simulink model "Dec_10_updated_33_bus_system_2MW_DG"  (R2023a)
settings: Solver=FixedStepAuto  StartTime=0.0  StopTime=0.3  RelTol=1e-3  EnableMultiTasking=on
undefined symbols (not defined in the file or in its folder): D1, Delta, DiscIntNeverNeededParam, Ts, Ts_Power
libraries: spsSeriesRLCBranchLib x42, spsThreePhaseVIMeasurementLib x35, spsThreePhaseSeriesRLCBranchLib x33, spsLoadFlowBusLib x33, spsThreePhaseParallelRLCLoadLib x31, simulink x8, spsMeanLib x5, spsFirstOrderFilterLib x4, spsStairGeneratorLib x3, spsBoostConverterLib x2, spsPowerPositiveSequenceLib x2, spsabctodq0Lib x2
(part 2 of 3)

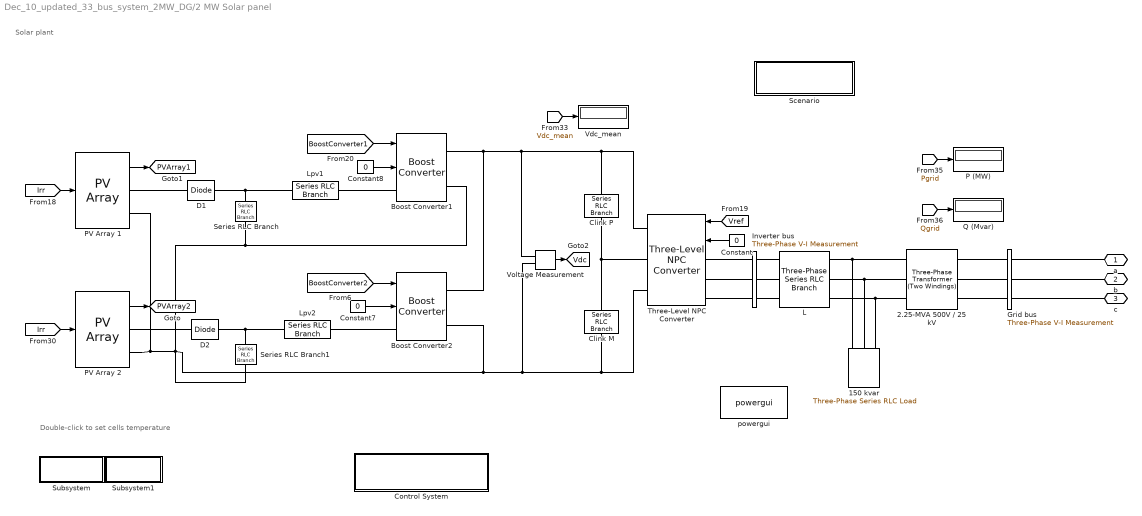
== system Dec_10_updated_33_bus_system_2MW_DG/2 MW Solar panel ==
  note: Solar plant
  note: Double-click to set cells temperature
  150 kvar : spsThreePhaseSeriesRLCLoadLib/Three-Phase Series RLC Load  LConnTagsString=A|B|C  Configuration=Y (grounded)  NominalVoltage=500  Vabc=[1e3 1e3 1e3]  Vabcp=[1e3 1e3 1e3]  NominalFrequency=50  UnbalancedPower=off  ActivePower=3000  InductivePower=0  CapacitivePower=150000  Pabc=[10e3 9e3 11e3]  QLabc=[100 90 110]  QCabc=[100 90 110]  Pabcp=[10e3 9e3 11e3]  QLabcp=[100 90 110]  QCabcp=[100 90 110]  Measurements=None  LoadType=constant Z
  2.25-MVA 500V / 25 kV : spsThreePhaseTransformerTwoWindingsLib/Three-Phase Transformer (Two Windings)  Winding1Connection=Yg  Winding2Connection=Delta (D1)  CoreType=Three single-phase transformers  SetSaturation=off  Hysteresis=off  DataFile='hysteresis'  SetInitialFlux=off  Measurements=None  UNITS=pu  NominalPower=[2.25e6 , 50 ]  Winding1=[ 33e3 , 0.001 , 0.03 ]  Winding2=[500 , 0.001 , 0.03 ]  Rm=200  Lm=200  L0=0.5  Saturation=[ 0,0 ; 0.0024,1.2 ; 1.0,1.52 ]  InitialFluxes=[ 0.8 , -0.8 , 0.7 ]  BreakLoop=off  DiscreteSolver=Trapezoidal iterative  DataType=off  TransfoNumber=0
  Boost Converter1 : spsBoostConverterLib/Boost Converter  ModelType=Switching devices  Ron=1e-4  Rs=1e6  Cs=inf  Vforward=[0,0]  Ron_Diode=1e-4  Rs_Diode=1e6  Cs_Diode=inf  Vf_Diode=0  Rs_CurrentSource=inf  Ron_ACsource=1e-3
      settings: LibrarySourceBlock=sps_lib/Power Electronics/Boost Converter
  Boost Converter2 : spsBoostConverterLib/Boost Converter  ModelType=Switching devices  Ron=1e-4  Rs=1e6  Cs=inf  Vforward=[0,0]  Ron_Diode=1e-4  Rs_Diode=1e6  Cs_Diode=inf  Vf_Diode=0  Rs_CurrentSource=inf  Ron_ACsource=1e-3
      settings: LibrarySourceBlock=sps_lib/Power Electronics/Boost Converter
  Clink M : spsSeriesRLCBranchLib/Series RLC Branch  LConnTagsString=__new0  RConnTagsString=__new0  BranchType=C  Resistance=1e-6  Inductance=1e-3  SetiL0=off  InitialCurrent=0  Capacitance=150e-3  Setx0=on  InitialVoltage=500  Measurements=None
  Clink P : spsSeriesRLCBranchLib/Series RLC Branch  LConnTagsString=__new0  RConnTagsString=__new0  BranchType=C  Resistance=1e-6  Inductance=1e-3  SetiL0=off  InitialCurrent=0  Capacitance=150e-3  Setx0=on  InitialVoltage=500  Measurements=None
  Constant : Constant  Value=0  SampleTime=Ts
  Constant7 : Constant  Value=0  SampleTime=Ts
  Constant8 : Constant  Value=0  SampleTime=Ts
  Control System : Subsystem
      mask Display: disp('CONTROL SYSTEM')
  D1 : spsDiodeLib/Diode  Ron=1e-4  Lon=0  Vf=0  IC=0  UseSnubber=0  Rs=1e6  Cs=inf  Measurements=off
  D2 : spsDiodeLib/Diode  Ron=1e-4  Lon=0  Vf=0  IC=0  UseSnubber=0  Rs=1e6  Cs=inf  Measurements=off
  Grid bus : spsThreePhaseVIMeasurementLib/Three-Phase V-I Measurement  VoltageMeasurement=phase-to-ground  SetLabelV=on  LabelV=Vgrid  Vpu=off  VpuLL=off  CurrentMeasurement=yes  SetLabelI=on  LabelI=Igrid  Ipu=off  Pbase=100e6  Vbase=500e3  OutputType=Magnitude  PhasorSimulation=off  PSBequivalent=0
  Inverter bus : spsThreePhaseVIMeasurementLib/Three-Phase V-I Measurement  VoltageMeasurement=phase-to-phase  SetLabelV=on  LabelV=Vinv  Vpu=off  VpuLL=off  CurrentMeasurement=no  SetLabelI=off  LabelI=Iabc_B1  Ipu=off  Pbase=100e6  Vbase=500e3  OutputType=Magnitude  PhasorSimulation=off  PSBequivalent=0
  L : spsThreePhaseSeriesRLCBranchLib/Three-Phase Series RLC Branch  LConnTagsString=A|B|C  RConnTagsString=A|B|C  BranchType=RL  Resistance=1e-3  Inductance=44.2e-6  Capacitance=inf  Measurements=None
  Lpv1 : spsSeriesRLCBranchLib/Series RLC Branch  LConnTagsString=__new0  RConnTagsString=__new0  BranchType=RL  Resistance=1e-3  Inductance=1e-3  SetiL0=off  InitialCurrent=0  Capacitance=120e-3  Setx0=off  InitialVoltage=0  Measurements=None
  Lpv2 : spsSeriesRLCBranchLib/Series RLC Branch  LConnTagsString=__new0  RConnTagsString=__new0  BranchType=RL  Resistance=1e-3  Inductance=1e-3  SetiL0=off  InitialCurrent=0  Capacitance=120e-3  Setx0=off  InitialVoltage=0  Measurements=None
  P (MW) : Display
      settings: Format=bank  Decimation=200
  PV Array 1 : spsPVArrayLib/PV Array  Npar=282  Nser=15  PlotType=array @ 1000 W/m2 & specified temperatures  S_vec=[ 1000 250]  Temp_C_vec="[ 45 25  ]"  ModuleName=User-defined  PlotWhenSelected=off  Pm=355.012  Ncell=83  Voc=51.9  Isc=8.68  Vm=43.4  Im=8.18  beta_Voc_pc=-0.304  alpha_Isc_pc=0.017  beta_Voc=-0.15778  alpha_Isc=0.0014756  IL=8.6865  I0=3.3093e-11  nI=0.92618  Rsh=389.4331  Rs=0.29289  RobustModel=on  RobustCellTemperature=25  BAL=on  Tc=1e-6  Tfilter=5e-5
      settings: AttributesFormatString=(%<RobustCellTemperature> deg. C)
  PV Array 2 : spsPVArrayLib/PV Array  Npar=122  Nser=14  PlotType=array @ 1000 W/m2 & specified temperatures  S_vec=[ 1000 250]  Temp_C_vec="[ 45 25  ]"  ModuleName=User-defined  PlotWhenSelected=off  Pm=293.664  Ncell=60  Voc=39.5  Isc=9.60  Vm=32.2  Im=9.12  beta_Voc_pc=-0.300  alpha_Isc_pc=0.03  beta_Voc=-0.1185  alpha_Isc=0.00288  IL=9.6627  I0=3.1923e-11  nI=0.96973  Rsh=336.4947  Rs=0.3029  RobustModel=on  RobustCellTemperature=25  BAL=on  Tc=1e-6  Tfilter=5e-5
      settings: AttributesFormatString=(%<RobustCellTemperature> deg. C)
  Q (Mvar) : Display
      settings: Format=bank  Decimation=200
  Scenario : Subsystem
      mask Display: disp('Scenario & Scopes')
  Series RLC Branch : spsSeriesRLCBranchLib/Series RLC Branch  LConnTagsString=__new0  RConnTagsString=__new0  BranchType=C  Resistance=1  Inductance=1e-3  SetiL0=off  InitialCurrent=0  Capacitance=200e-6  Setx0=on  InitialVoltage=650  Measurements=None
  Series RLC Branch1 : spsSeriesRLCBranchLib/Series RLC Branch  LConnTagsString=__new0  RConnTagsString=__new0  BranchType=C  Resistance=1  Inductance=1e-3  SetiL0=off  InitialCurrent=0  Capacitance=200e-6  Setx0=on  InitialVoltage=450  Measurements=None
  Subsystem : Subsystem
      settings: OpenFcn=|
      | SystemName1=gcs;
      | BlockName1=[SystemName1, '/', 'PV Array 1'];
      | set_param(BlockName1,'RobustCellTemperature','25');
      | set_param(BlockName1,'ForegroundColor','black');
      | BlockName2=[SystemName1, '/', 'PV Array 2'];
      | set_param(BlockName2,'RobustCellTemperature','25');
      | set_param(BlockName2,'ForegroundColor','black');
      mask Display: disp('25 deg. C')
  Subsystem1 : Subsystem
      settings: OpenFcn=|
      | SystemName1=gcs;
      | BlockName1=[SystemName1, '/', 'PV Array 1'];
      | set_param(BlockName1,'RobustCellTemperature','45');
      | set_param(BlockName1,'ForegroundColor','red');
      | BlockName2=[SystemName1, '/', 'PV Array 2'];
      | set_param(BlockName2,'RobustCellTemperature','45');
      | set_param(BlockName2,'ForegroundColor','red');
      mask Display: disp('45 deg. C')
  Three-Level NPC Converter : spsThreeLevelNPCConverterLib/Three-Level NPC Converter  ModelType=Switching devices  Ron=1e-4/2  Rs=1e6  Cs=inf  Vforward=[0,0]  Ron_Diode=1e-4  Rs_Diode=1e6  Cs_Diode=inf  Vf_Diode=0  Rs_CurrentSource=inf  Ron_ACsource=1e-3
      settings: LibrarySourceBlock=|
      | sps_lib/Power Electronics/Three-Level
      | NPC Converter
  Vdc_mean : Display
      settings: Decimation=200
  Voltage Measurement : spsVoltageMeasurementLib/Voltage Measurement  PhasorSimulation=off  OutputType=Complex  PSBequivalent=0
  powergui : spspowerguiLib/powergui  Priority=2  SimulationMode=Discrete  SampleTime=Ts_Power  frequency=60  Iterations=50  frequencyindice=0  Pbase=100e6  ErrMax=1e-4  UnitsV=kV  UnitsW=MW  buscounter=0  FunctionMessages=off  echomessages=off  EnableUseOfTLC=off  CurrentSourceSwitches=off  DisableSnubberDevices=off  DisableRonSwitches=off  DisableVfSwitches=off  DisplayEquations=off  AutomaticDiscreteSolvers=off  SolverType=Tustin/Backward Euler (TBE)  Interpol=off  ExternalGateDelay=off  methode=off  Ts=0  x0status=blocks  SPID=off  SwTol=0  HookPort=off  NonlinearTolerance=1e-4  nMaxIteration=100  ContinueOnMaxIteration=on  RestoreLinks=warning  ResistiveCurrentMeasurement=off  Frange=[0:2:500]  Ylog=off  Xlog=off  ShowGrid=off  save=off  variable=ZData  structure=Scope_VIgrid  ZoomFFT=off  StartTime=0.18  cycles=1  DisplayStyle=1  fundamental=60  FreqAxis=on  MaxFrequency=3500  frequencyindicesteady=1  RmsSteady=1  display=off
  a : PMIOPort  Side=Right
  b : PMIOPort  Port=2  Side=Right
  c : PMIOPort  Port=3  Side=Right
  tag scope: PVArray1=global, PVArray2=global, Vdc=global
  wires:
  [Pgrid] -> P (MW)/1
  Constant7/1 -> Boost Converter2/2
  Constant8/1 -> Boost Converter1/2
  PV Array 2/1 -> [PVArray2]
  PV Array 1/1 -> [PVArray1]
  [Irr] -> PV Array 2/1
  [BoostConverter1] -> Boost Converter1/1
  Constant/1 -> Three-Level NPC Converter/2
  [Vdc_mean] -> Vdc_mean/1
  [Vref] -> Three-Level NPC Converter/1
  [BoostConverter2] -> Boost Converter2/1
  Voltage Measurement/1 -> [Vdc]
  [Qgrid] -> Q (Mvar)/1
  [Irr] -> PV Array 1/1
  connections:
  Series RLC Branch/RConn1 -- Boost Converter1/RConn2 -- Boost Converter2/RConn2 -- Clink M/RConn1 -- Three-Level NPC Converter/RConn3 -- Voltage Measurement/LConn2 -- Series RLC Branch1/RConn1 -- PV Array 2/RConn2 -- PV Array 1/RConn2
  Inverter bus/RConn1 -- L/LConn1
  PV Array 1/RConn1 -- D1/LConn1
  Grid bus/LConn1 -- 2.25-MVA 500V / 25 kV/LConn1
  Lpv1/LConn1 -- Boost Converter1/LConn1
  c/RConn1 -- Grid bus/RConn3
  Inverter bus/RConn3 -- L/LConn3
  D2/LConn1 -- PV Array 2/RConn1
  Three-Level NPC Converter/LConn3 -- Inverter bus/LConn3
  Lpv2/RConn1 -- D2/RConn1 -- Series RLC Branch1/LConn1
  Lpv2/LConn1 -- Boost Converter2/LConn1
  Grid bus/LConn2 -- 2.25-MVA 500V / 25 kV/LConn2
  a/RConn1 -- Grid bus/RConn1
  Grid bus/LConn3 -- 2.25-MVA 500V / 25 kV/LConn3
  2.25-MVA 500V / 25 kV/RConn2 -- 150 kvar/LConn2 -- L/RConn2
  2.25-MVA 500V / 25 kV/RConn1 -- 150 kvar/LConn1 -- L/RConn1
  b/RConn1 -- Grid bus/RConn2
  Boost Converter1/RConn1 -- Boost Converter2/RConn1 -- Three-Level NPC Converter/RConn1 -- Clink P/LConn1 -- Voltage Measurement/LConn1
  Three-Level NPC Converter/LConn2 -- Inverter bus/LConn2
  2.25-MVA 500V / 25 kV/RConn3 -- 150 kvar/LConn3 -- L/RConn3
  Lpv1/RConn1 -- D1/RConn1 -- Series RLC Branch/LConn1
  Three-Level NPC Converter/LConn1 -- Inverter bus/LConn1
  Clink M/LConn1 -- Clink P/RConn1 -- Three-Level NPC Converter/RConn2
  Inverter bus/RConn2 -- L/LConn2

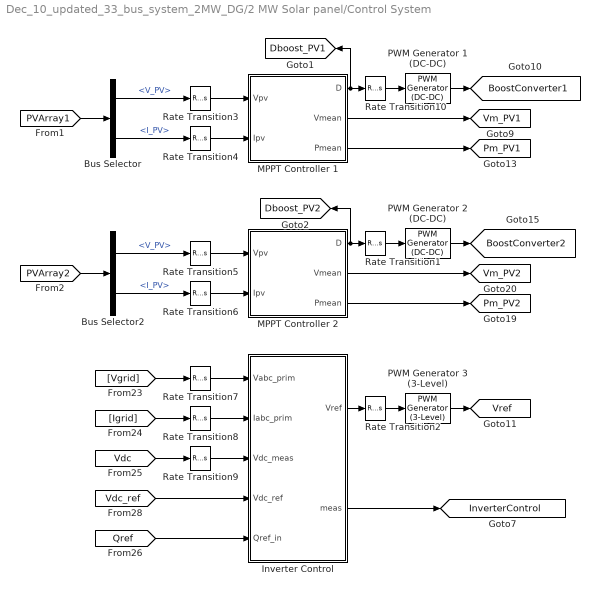
== system Dec_10_updated_33_bus_system_2MW_DG/2 MW Solar panel/Control System ==
  Bus Selector : BusSelector  OutputSignals=V_PV,I_PV
  Bus Selector2 : BusSelector  OutputSignals=V_PV,I_PV
  Inverter Control : Subsystem  mask(Inverter Control){Pnom=2.25e6, Fnom=50, Vnom_prim=33e3, Vnom_sec=500, Vnom_dc=1000, Kp_Preg=1, Ki_Preg=75, Kp_VDCreg=10, Ki_VDCreg=500, Kp_Ireg=0.3, Ki_Ireg=20, RLff=[ 0.004, 0.21], Ts=Ts}
      mask prompts: Pnom "Power (VA)"; Fnom "Frequency (Hz)"; Vnom_prim "Primary voltage (Vrms)"; Vnom_sec "Secondary voltage (Vrms)"; Vnom_dc "DC voltage (V)"; Kp_Preg "Proportional gain"; Ki_Preg "Integral gain"; Kp_VDCreg "Proportional gain"; Ki_VDCreg "Integral gain"; Kp_Ireg "Proportional gain"; Ki_Ireg "Integral gain"; RLff "Feedforward Values [Rff Lff] (pu)"; Ts "Control sample time:"
      mask help: Control system for a 2-MW, 1-Mvar, 25-kV, Grid-Connected Inverter
      mask init:
      | Rff=RLff(1);
      | Lff=RLff(2);
      | Limits_Ireg=[1.5, -1.5];
      | Limits_VDCreg=[1.5, -1.5];
      | Limits_Preg=[1.5, -1.5];
      | Limits_Qreg=[1.5, -1.5];
      mask DialogControl Container4 Prompt: Nominal Values:
      mask DialogControl Container16 Prompt: Power regulators
      mask DialogControl Container8 Prompt: Voltage regulator:
      mask DialogControl Container6 Prompt: Current regulators:
      mask DialogControl Ts1 Prompt: Sample time (s)
  MPPT Controller 1 : Subsystem  mask(MPPT Controller - Perturb and Observe algorithm (PandO)){Dinit=0.35, Dlimits=[0.8, 0.3], deltaD=60e-6, Fc=1000, Ts=Ts}
      mask prompts: Dinit "Duty cycle (D) initial value"; Dlimits "D limits [Upper, Lower]"; deltaD "Increment value for PandO algorithm"; Fc "Measurement filter cutoff frequency (Hz)"; Ts "Sample time (s)"
      mask init:
      | Dmax=Dlimits(1);
      | Dmin=Dlimits(2);
  MPPT Controller 2 : Subsystem  mask(MPPT Controller - Perturb and Observe algorithm (PandO)){Dinit=0.55, Dlimits=[0.8, 0.47], deltaD=60e-6, Fc=1000, Ts=Ts}
      mask prompts: Dinit "Duty cycle (D) initial value"; Dlimits "D limits [Upper, Lower]"; deltaD "Increment value for PandO algorithm"; Fc "Measurement filter cutoff frequency (Hz)"; Ts "Sample time (s)"
      mask init:
      | Dmax=Dlimits(1);
      | Dmin=Dlimits(2);
  PWM Generator 1 (DC-DC) : spsPWMGeneratorDCDCLib/PWM Generator (DC-DC)  Fsw=5000  Ts=Ts_Power
  PWM Generator 2 (DC-DC) : spsPWMGeneratorDCDCLib/PWM Generator (DC-DC)  Fsw=5000  Ts=Ts_Power
  PWM Generator 3 (3-Level) : spsPWMGenerator3LevelLib/PWM Generator (3-Level)  ModulatorType=Three-phase bridge (12 pulses)  ModulatorMode=Unsynchronized  nF=27  Fc=39*60  ModulatingSignals=off  m=0.8  Freq=60  Phase=0  Ts=Ts_Power
      settings: LibrarySourceBlock=|
      | sps_lib/Power Electronics/Power Electronics Control/PWM Generator
      | (3-Level)
  Rate Transition1 : RateTransition  OutPortSampleTime=Ts_Power
  Rate Transition10 : RateTransition  OutPortSampleTime=Ts_Power
  Rate Transition2 : RateTransition  OutPortSampleTime=Ts_Power
  Rate Transition{3..9} (7 alike) : RateTransition  OutPortSampleTime=Ts
  tag scope: BoostConverter1=global, BoostConverter2=global, Dboost_PV1=global, Dboost_PV2=global, InverterControl=global, Pm_PV1=global, Pm_PV2=global, Vm_PV1=global, Vm_PV2=global, Vref=global
  wires:
  Inverter Control/1(Vref) -> Rate Transition2/1
  MPPT Controller 2/2(Vmean) -> [Vm_PV2]
  [Vgrid] -> Rate Transition7/1
  [Vdc_ref] -> Inverter Control/4(Vdc_ref)
  Bus Selector2/1 -> Rate Transition5/1  "<V_PV>"
  Rate Transition3/1 -> MPPT Controller 1/1(Vpv)
  Rate Transition2/1 -> PWM Generator 3 (3-Level)/1
  Rate Transition4/1 -> MPPT Controller 1/2(Ipv)
  [Igrid] -> Rate Transition8/1
  Bus Selector/2 -> Rate Transition4/1  "<I_PV>"
  MPPT Controller 2/3(Pmean) -> [Pm_PV2]
  [Qref] -> Inverter Control/5(Qref_in)
  [Vdc] -> Rate Transition9/1
  MPPT Controller 1/1(D) -> [Dboost_PV1], Rate Transition10/1
  Bus Selector/1 -> Rate Transition3/1  "<V_PV>"
  Bus Selector2/2 -> Rate Transition6/1  "<I_PV>"
  Rate Transition1/1 -> PWM Generator 2 (DC-DC)/1
  Rate Transition6/1 -> MPPT Controller 2/2(Ipv)
  Rate Transition8/1 -> Inverter Control/2(Iabc_prim)
  Rate Transition7/1 -> Inverter Control/1(Vabc_prim)
  MPPT Controller 1/3(Pmean) -> [Pm_PV1]
  MPPT Controller 1/2(Vmean) -> [Vm_PV1]
  Rate Transition9/1 -> Inverter Control/3(Vdc_meas)
  Rate Transition10/1 -> PWM Generator 1 (DC-DC)/1
  MPPT Controller 2/1(D) -> [Dboost_PV2], Rate Transition1/1
  Rate Transition5/1 -> MPPT Controller 2/1(Vpv)
  PWM Generator 1 (DC-DC)/1 -> [BoostConverter1]
  PWM Generator 2 (DC-DC)/1 -> [BoostConverter2]
  Inverter Control/2(meas) -> [InverterControl]
  PWM Generator 3 (3-Level)/1 -> [Vref]
  [PVArray1] -> Bus Selector/1
  [PVArray2] -> Bus Selector2/1

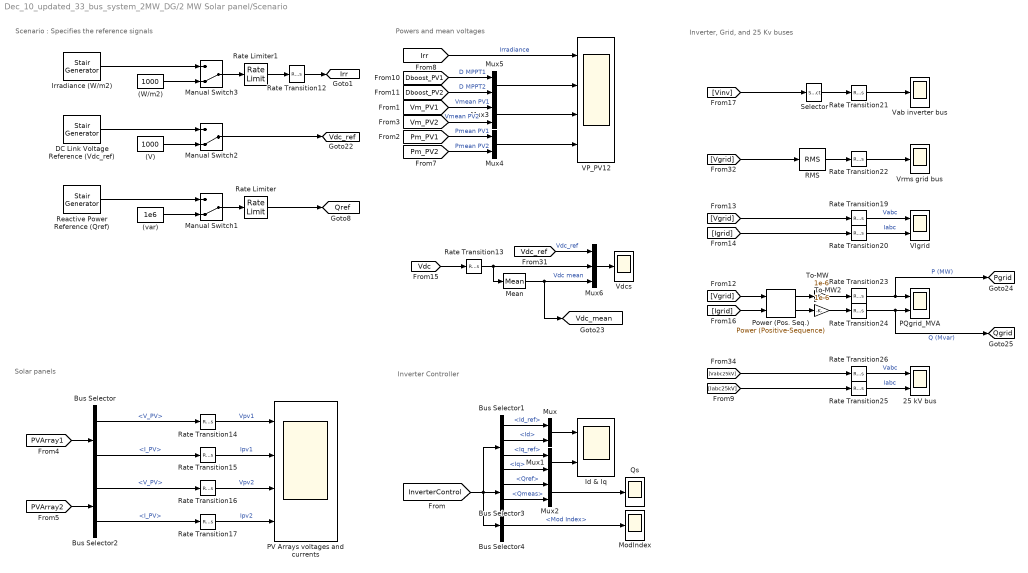
== system Dec_10_updated_33_bus_system_2MW_DG/2 MW Solar panel/Scenario ==
  note: Powers and mean voltages
  note: Inverter, Grid, and 25 Kv buses
  note: Inverter Controller
  note: Solar panels
  note: Scenario : Specifies the reference signals
  (V) : Constant  Value=1000
  (W/m2) : Constant  Value=1000
  (var) : Constant  Value=1e6
  25 kV bus : Scope  NumInputPorts=2
  Bus Selector : BusSelector  OutputSignals=V_PV,I_PV
  Bus Selector1 : BusSelector  OutputSignals=Id_ref,Id,Iq_ref,Iq
  Bus Selector2 : BusSelector  OutputSignals=V_PV,I_PV
  Bus Selector3 : BusSelector  OutputSignals=Qref,Qmeas
  Bus Selector4 : BusSelector  OutputSignals=Mod Index
  DC Link Voltage Reference (Vdc_ref) : spsStairGeneratorLib/Stair Generator  t=[0, 0.2, 0.4]  e=[1000, 1050, 1000]  Ts=Ts
  Id & Iq : Scope  NumInputPorts=2
  Irradiance (W/m2) : spsStairGeneratorLib/Stair Generator  t=[0, 0.2, 0.4]  e=[1000, 250,1000]  Ts=Ts
  Manual Switch1 : ManualSwitch  CurrentSetting=0
  Manual Switch2 : ManualSwitch  CurrentSetting=0
  Manual Switch3 : ManualSwitch  CurrentSetting=0
  Mean : spsMeanLib/Mean  Freq=50  Vinit=1000  Ts=Ts
  ModIndex : Scope
  Mux{,1..5} (6 alike) : Mux  Inputs=2
  Mux6 : Mux  Inputs=3
  PQgrid_MVA : Scope  NumInputPorts=2
  PV Arrays voltages and currents : Scope  NumInputPorts=4
  Power (Pos. Seq.) : spsPowerPositiveSequenceLib/Power (Positive-Sequence)  Freq=60  Vinit=[20570,-37]  Iinit=[70, -63]  Ts=Ts_Power
      settings: LibrarySourceBlock=|
      | sps_lib/Sensors and Measurements/Power
      | (Positive-Sequence)
  Qs : Scope
  RMS : spsRMSLib/RMS  TrueRMS=off  Freq=60  RMSInit=25000  Ts=Ts_Power
  Rate Limiter : RateLimiter  RisingSlewLimit=1e6/(1/60)  FallingSlewLimit=-1e6/(1/60)  SampleTimeMode=inherited  InitialCondition=1e6
  Rate Limiter1 : RateLimiter  RisingSlewLimit=1000/(1/60)  FallingSlewLimit=-1000/(1/60)  SampleTimeMode=inherited  InitialCondition=1000
  Rate Transition12 : RateTransition  OutPortSampleTime=Ts_Power
  Rate Transition{13..17,19..26} (13 alike) : RateTransition  OutPortSampleTime=Ts
  "Reactive Power Reference (Qref) " : spsStairGeneratorLib/Stair Generator  t=[0, 0.2, 0.4]  e=[1e6, -1e6, 1e6]  Ts=Ts
  Selector : Selector  InputPortWidth=3  IndexOptions=Index vector (dialog)  Indices=1  OutputSizes=1
  To-MW : Gain  Gain=1e-6
  To-MW2 : Gain  Gain=1e-6
  VIgrid : Scope  NumInputPorts=2
  VP_PV12 : Scope  NumInputPorts=4
  Vab inverter bus : Scope
  Vdcs : Scope
  Vrms grid bus : Scope
  tag scope: Irr=global, Pgrid=global, Qgrid=global, Qref=global, Vdc_mean=global, Vdc_ref=global
  wires:
  Rate Limiter/1 -> [Qref]
  (W/m2)/1 -> Manual Switch3/2
  (V)/1 -> Manual Switch2/2
  DC Link Voltage Reference (Vdc_ref)/1 -> Manual Switch2/1
  Rate Limiter1/1 -> Rate Transition12/1
  (var)/1 -> Manual Switch1/2
  "Reactive Power Reference (Qref) "/1 -> Manual Switch1/1
  Manual Switch1/1 -> Rate Limiter/1
  Manual Switch2/1 -> [Vdc_ref]
  Irradiance (W/m2)/1 -> Manual Switch3/1
  Manual Switch3/1 -> Rate Limiter1/1
  Rate Transition12/1 -> [Irr]
  Bus Selector2/1 -> Rate Transition16/1  "<V_PV>"
  Bus Selector/2 -> Rate Transition15/1  "<I_PV>"
  Bus Selector/1 -> Rate Transition14/1  "<V_PV>"
  Rate Transition19/1 -> VIgrid/1  "Vabc"
  [Pm_PV1] -> Mux4/1  "Pmean PV1"
  Rate Transition17/1 -> PV Arrays voltages and currents/4  "Ipv2"
  RMS/1 -> Rate Transition22/1
  [Pm_PV2] -> Mux4/2  "Pmean PV2"
  [Irr] -> VP_PV12/1  "Irradiance"
  Rate Transition22/1 -> Vrms grid bus/1
  Rate Transition16/1 -> PV Arrays voltages and currents/3  "Vpv2"
  Rate Transition26/1 -> 25 kV bus/1  "Vabc"
  Mux3/1 -> VP_PV12/3
  [Vgrid] -> RMS/1
  [Vgrid] -> Power (Pos. Seq.)/1
  Rate Transition23/1 -> [Pgrid], PQgrid_MVA/1  "P (MW)"
  [PVArray1] -> Bus Selector/1
  Rate Transition20/1 -> VIgrid/2  "Iabc"
  Bus Selector1/2 -> Mux/2  "<Id>"
  Mux6/1 -> Vdcs/1
  Bus Selector1/1 -> Mux/1  "<Id_ref>"
  Mux4/1 -> VP_PV12/4
  Rate Transition15/1 -> PV Arrays voltages and currents/2  "Ipv1"
  Bus Selector1/3 -> Mux1/1  "<Iq_ref>"
  Mux5/1 -> VP_PV12/2
  Power (Pos. Seq.)/2 -> To-MW2/1
  [Igrid] -> Rate Transition20/1
  [Vabc25kV] -> Rate Transition26/1
  Mux1/1 -> Id & Iq/2
  Mux/1 -> Id & Iq/1
  Rate Transition25/1 -> 25 kV bus/2  "Iabc"
  Bus Selector3/2 -> Mux2/2  "<Qmeas>"
  [Vm_PV2] -> Mux3/2  "Vmean PV2"
  Rate Transition14/1 -> PV Arrays voltages and currents/1  "Vpv1"
  Mux2/1 -> Qs/1
  [Vgrid] -> Rate Transition19/1
  Rate Transition13/1 -> Mean/1, Mux6/2
  Power (Pos. Seq.)/1 -> To-MW/1
  [Dboost_PV1] -> Mux5/1  "D MPPT1"
  Bus Selector4/1 -> ModIndex/1  "<Mod Index>"
  Bus Selector3/1 -> Mux2/1  "<Qref>"
  [InverterControl] -> Bus Selector1/1, Bus Selector4/1, Bus Selector3/1
  [Vinv] -> Selector/1
  Mean/1 -> Mux6/3, [Vdc_mean]  "Vdc mean"
  [Dboost_PV2] -> Mux5/2  "D MPPT2"
  [Vm_PV1] -> Mux3/1  "Vmean PV1"
  [Vdc_ref] -> Mux6/1  "Vdc_ref"
  Bus Selector1/4 -> Mux1/2  "<Iq>"
  [Igrid] -> Power (Pos. Seq.)/2
  Bus Selector2/2 -> Rate Transition17/1  "<I_PV>"
  [Iabc25kV] -> Rate Transition25/1
  Rate Transition24/1 -> [Qgrid], PQgrid_MVA/2  "Q (Mvar)"
  [Vdc] -> Rate Transition13/1
  [PVArray2] -> Bus Selector2/1
  Selector/1 -> Rate Transition21/1
  Rate Transition21/1 -> Vab inverter bus/1
  To-MW2/1 -> Rate Transition24/1
  To-MW/1 -> Rate Transition23/1

== system Dec_10_updated_33_bus_system_2MW_DG/2 MW Solar panel/Subsystem ==

== system Dec_10_updated_33_bus_system_2MW_DG/2 MW Solar panel/Subsystem1 ==

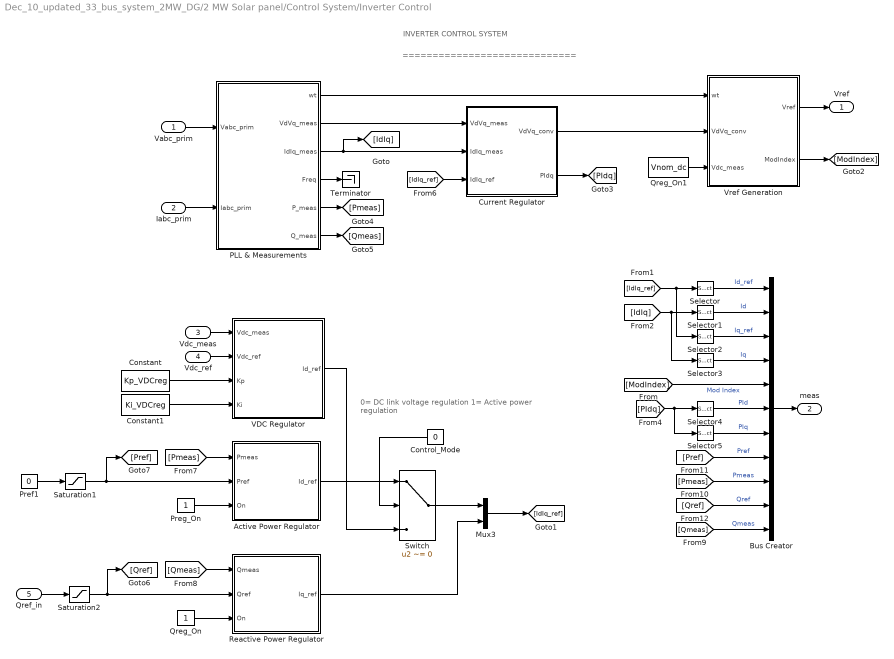
== system Dec_10_updated_33_bus_system_2MW_DG/2 MW Solar panel/Control System/Inverter Control ==
  note: INVERTER CONTROL SYSTEM
  note: =============================
  note: 0= DC link voltage regulation
      | 1= Active power regulation
  Vabc_prim : Inport  PortDimensions=3
  Iabc_prim : Inport  Port=2  PortDimensions=3
  Vdc_meas : Inport  Port=3  PortDimensions=1
  Vdc_ref : Inport  Port=4  PortDimensions=1
  Qref_in : Inport  Port=5  PortDimensions=1
  Active Power Regulator : Subsystem
  Bus Creator : BusCreator  Inputs=11
  Constant : Constant  Value=Kp_VDCreg  SampleTime=Ts
  Constant1 : Constant  Value=Ki_VDCreg  SampleTime=Ts
  Control_Mode : Constant  Value=0
  Current Regulator : Subsystem
  Mux3 : Mux  Inputs=2
  PLL & Measurements : Subsystem
  Pref1 : Constant  Value=0  SampleTime=Ts
  Preg_On : Constant
  Qreg_On : Constant
  Qreg_On1 : Constant  Value=Vnom_dc
  Reactive Power Regulator : Subsystem
  Saturation1 : Saturate  UpperLimit=2e6  LowerLimit=-2e6
  Saturation2 : Saturate  UpperLimit=1e6  LowerLimit=-1e6
  Selector : Selector  InputPortWidth=2  IndexOptions=Index vector (dialog)  Indices=1  OutputSizes=1
  Selector1 : Selector  InputPortWidth=2  IndexOptions=Index vector (dialog)  Indices=1  OutputSizes=1
  Selector2 : Selector  InputPortWidth=2  IndexOptions=Index vector (dialog)  Indices=2  OutputSizes=1
  Selector3 : Selector  InputPortWidth=2  IndexOptions=Index vector (dialog)  Indices=2  OutputSizes=1
  Selector4 : Selector  InputPortWidth=2  IndexOptions=Index vector (dialog)  Indices=1  OutputSizes=1
  Selector5 : Selector  InputPortWidth=2  IndexOptions=Index vector (dialog)  Indices=2  OutputSizes=1
  Switch : Switch  Criteria=u2 ~= 0  SaturateOnIntegerOverflow=off  InputSameDT=off
  Terminator : Terminator
  VDC Regulator : Subsystem
  Vref Generation : Subsystem
  Vref : Outport  VectorParamsAs1DForOutWhenUnconnected=off
  meas : Outport  Port=2  VectorParamsAs1DForOutWhenUnconnected=off
  wires:
  Constant/1 -> VDC Regulator/3(Kp)
  Control_Mode/1 -> Switch/2
  Active Power Regulator/1(Id_ref) -> Switch/1
  VDC Regulator/1(Id_ref) -> Switch/3
  Current Regulator/1(VdVq_conv) -> Vref Generation/2(VdVq_conv)
  Qreg_On/1 -> Reactive Power Regulator/3(On)
  PLL & Measurements/1(wt) -> Vref Generation/1(wt)
  Selector3/1 -> Bus Creator/4  "Iq"
  PLL & Measurements/2(VdVq_meas) -> Current Regulator/1(VdVq_meas)
  [ModIndex] -> Bus Creator/5  "Mod Index"
  [IdIq_ref] -> Selector/1, Selector2/1
  Pref1/1 -> Saturation1/1
  PLL & Measurements/5(P_meas) -> [Pmeas]
  Current Regulator/2(PIdq) -> [PIdq]
  Vabc_prim/1 -> PLL & Measurements/1(Vabc_prim)
  Mux3/1 -> [IdIq_ref]
  [Pmeas] -> Bus Creator/9  "Pmeas"
  Reactive Power Regulator/1(Iq_ref) -> Mux3/2
  [PIdq] -> Selector5/1, Selector4/1
  [IdIq_ref] -> Current Regulator/3(IdIq_ref)
  [Qmeas] -> Reactive Power Regulator/1(Qmeas)
  PLL & Measurements/6(Q_meas) -> [Qmeas]
  Selector2/1 -> Bus Creator/3  "Iq_ref"
  [Pmeas] -> Active Power Regulator/1(Pmeas)
  [Qref] -> Bus Creator/10  "Qref"
  [Pref] -> Bus Creator/8  "Pref"
  Selector/1 -> Bus Creator/1  "Id_ref"
  [Qmeas] -> Bus Creator/11  "Qmeas"
  PLL & Measurements/3(IdIq_meas) -> Current Regulator/2(IdIq_meas), [IdIq]
  Vdc_ref/1 -> VDC Regulator/2(Vdc_ref)
  [IdIq] -> Selector1/1, Selector3/1
  Preg_On/1 -> Active Power Regulator/3(On)
  Switch/1 -> Mux3/1
  Vref Generation/2(ModIndex) -> [ModIndex]
  Iabc_prim/1 -> PLL & Measurements/2(Iabc_prim)
  PLL & Measurements/4(Freq) -> Terminator/1
  Vref Generation/1(Vref) -> Vref/1
  Selector4/1 -> Bus Creator/6  "PId"
  Vdc_meas/1 -> VDC Regulator/1(Vdc_meas)
  Selector5/1 -> Bus Creator/7  "PIq"
  Selector1/1 -> Bus Creator/2  "Id"
  Qreg_On1/1 -> Vref Generation/3(Vdc_meas)
  Qref_in/1 -> Saturation2/1
  Saturation2/1 -> [Qref], Reactive Power Regulator/2(Qref)
  Constant1/1 -> VDC Regulator/4(Ki)
  Bus Creator/1 -> meas/1
  Saturation1/1 -> [Pref], Active Power Regulator/2(Pref)

== system Dec_10_updated_33_bus_system_2MW_DG/2 MW Solar panel/Control System/MPPT Controller 1 ==
  Vpv : Inport
  Ipv : Inport  Port=2
  First-Order Filter : spsFirstOrderFilterLib/First-Order Filter  FilterType=Lowpass  Tc=1/Fc  Ts=Ts  Initialize=off  Vac_Init=[0, 0, 60]  Vdc_Init=0  PlotResponse=off  FreqRange="[0,  200,  1]"
  First-Order Filter1 : spsFirstOrderFilterLib/First-Order Filter  FilterType=Lowpass  Tc=1/Fc  Ts=Ts  Initialize=off  Vac_Init=[0, 0, 60]  Vdc_Init=0  PlotResponse=off  FreqRange="[0,  200,  1]"
  "MPPT Control 1 " : MATLAB Function  TreatAsAtomicUnit=on
  Mean1 : spsMeanLib/Mean  Freq=50  Vinit=650  Ts=Ts
  Mean2 : spsMeanLib/Mean  Freq=50  Vinit=1500e3  Ts=Ts
  Product1 : Product
  D : Outport  VectorParamsAs1DForOutWhenUnconnected=off
  Vmean : Outport  Port=2  VectorParamsAs1DForOutWhenUnconnected=off
  Pmean : Outport  Port=3  VectorParamsAs1DForOutWhenUnconnected=off
  wires:
  First-Order Filter1/1 -> "MPPT Control 1 "/2(I)
  First-Order Filter/1 -> "MPPT Control 1 "/1(V)
  Ipv/1 -> Product1/2, First-Order Filter1/1
  Vpv/1 -> Mean1/1, Product1/1, First-Order Filter/1
  "MPPT Control 1 "/1(D) -> D/1
  Product1/1 -> Mean2/1
  Mean1/1 -> Vmean/1
  Mean2/1 -> Pmean/1

== system Dec_10_updated_33_bus_system_2MW_DG/2 MW Solar panel/Control System/MPPT Controller 2 ==
  Vpv : Inport
  Ipv : Inport  Port=2
  First-Order Filter : spsFirstOrderFilterLib/First-Order Filter  FilterType=Lowpass  Tc=1/Fc  Ts=Ts  Initialize=off  Vac_Init=[0, 0, 60]  Vdc_Init=0  PlotResponse=off  FreqRange="[0,  200,  1]"
  First-Order Filter1 : spsFirstOrderFilterLib/First-Order Filter  FilterType=Lowpass  Tc=1/Fc  Ts=Ts  Initialize=off  Vac_Init=[0, 0, 60]  Vdc_Init=0  PlotResponse=off  FreqRange="[0,  200,  1]"
  "MPPT Control 1 " : MATLAB Function  TreatAsAtomicUnit=on
  Mean1 : spsMeanLib/Mean  Freq=50  Vinit=420  Ts=Ts
  Mean2 : spsMeanLib/Mean  Freq=50  Vinit=500e3  Ts=Ts
  Product1 : Product
  D : Outport  VectorParamsAs1DForOutWhenUnconnected=off
  Vmean : Outport  Port=2  VectorParamsAs1DForOutWhenUnconnected=off
  Pmean : Outport  Port=3  VectorParamsAs1DForOutWhenUnconnected=off
  wires:
  "MPPT Control 1 "/1(D) -> D/1
  Ipv/1 -> Product1/2, First-Order Filter1/1
  First-Order Filter/1 -> "MPPT Control 1 "/1(V)
  First-Order Filter1/1 -> "MPPT Control 1 "/2(I)
  Mean1/1 -> Vmean/1
  Product1/1 -> Mean2/1
  Mean2/1 -> Pmean/1
  Vpv/1 -> Product1/1, Mean1/1, First-Order Filter/1

== system Dec_10_updated_33_bus_system_2MW_DG/2 MW Solar panel/Control System/Inverter Control/Active Power Regulator ==
  Pmeas : Inport  PortDimensions=1
  Pref : Inport  Port=2  PortDimensions=1
  On : Inport  Port=3  PortDimensions=1
  Constant1 : Constant  Value=0
  Constant2 : Constant
  PI regulator with anti-windup D : Subsystem  DialogController=POWERSYS.PowerSysDialog  mask(Discrete PI Controller){Kp=Kp_Preg, Ki=Ki_Preg, Par_Limits=Limits_Preg, Init=0, Ts=Ts}
      mask prompts: Kp "Proportional gain (Kp):"; Ki "Integral gain (Ki):"; Par_Limits "Output limits: [ Upper   Lower ]"; Init "Output initial value:"; Ts "Sample time:"
      mask help: This block implements a discrete PI controller.
      mask init:
      | UpperLimit=Par_Limits(1);
      | LowerLimit=Par_Limits(2);
      | power_initmask();
      mask Help: This block is part of a subset of blocks in the Extras library that does not have documentation associated with it, other than the block mask description.
      mask Display: disp('PI');
  Sum : Sum  Inputs=|+-
  Switch : Switch  Criteria=u2 ~= 0  SaturateOnIntegerOverflow=off  InputSameDT=off
  W->pu1 : Gain  Gain=1/Pnom  SaturateOnIntegerOverflow=on  OutDataTypeStr=Inherit: Same as input  ParamDataTypeStr=Inherit: Same as input
  Id_ref : Outport  InitialOutput=0  VectorParamsAs1DForOutWhenUnconnected=off
  wires:
  W->pu1/1 -> PI regulator with anti-windup D/1(Error)
  Sum/1 -> W->pu1/1
  Pmeas/1 -> Sum/2
  Pref/1 -> Sum/1
  PI regulator with anti-windup D/1(Out) -> Id_ref/1
  Constant2/1 -> Switch/3
  Switch/1 -> PI regulator with anti-windup D/2(Reset)
  On/1 -> Switch/2
  Constant1/1 -> Switch/1

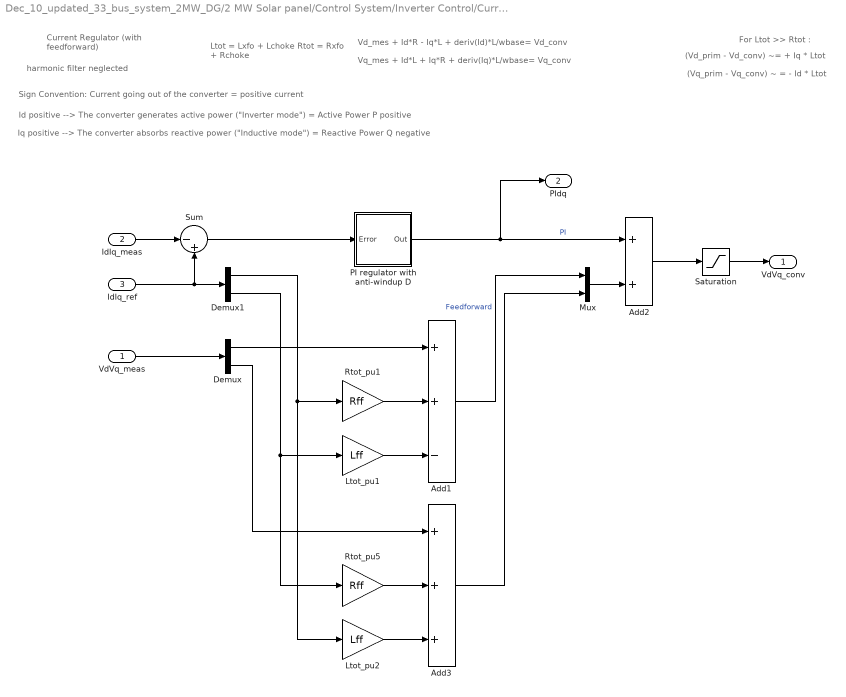
== system Dec_10_updated_33_bus_system_2MW_DG/2 MW Solar panel/Control System/Inverter Control/Current Regulator ==
  note: harmonic filter neglected
  note: Vd_mes + Id*R - Iq*L + deriv(Id)*L/wbase= Vd_conv
  note: Vq_mes + Id*L + Iq*R + deriv(Iq)*L/wbase= Vq_conv
  note: Current Regulator
      | (with feedforward)
  note: Sign Convention: Current going out of the converter = positive current
  note: Iq positive --> The converter absorbs reactive power ("Inductive mode") = Reactive Power Q negative
  note: Id positive --> The converter generates active power ("Inverter mode") = Active Power P positive
  note: Ltot = Lxfo + Lchoke
      | Rtot = Rxfo + Rchoke
  note: (Vd_prim - Vd_conv) ~= + Iq * Ltot
  note: (Vq_prim - Vq_conv) ~ = - Id * Ltot
  note: For Ltot >> Rtot :
  VdVq_meas : Inport  PortDimensions=2
  IdIq_meas : Inport  Port=2  PortDimensions=2
  IdIq_ref : Inport  Port=3  PortDimensions=2
  Add1 : Sum  Inputs=++-
  Add2 : Sum
  Add3 : Sum  Inputs=+++
  Demux : Demux  Outputs=2
  Demux1 : Demux  Outputs=2
  Ltot_pu1 : Gain  Gain=Lff  SaturateOnIntegerOverflow=on  OutDataTypeStr=Inherit: Same as input  ParamDataTypeStr=Inherit: Same as input
  Ltot_pu2 : Gain  Gain=Lff  SaturateOnIntegerOverflow=on  OutDataTypeStr=Inherit: Same as input  ParamDataTypeStr=Inherit: Same as input
  Mux : Mux  Inputs=2
  PI regulator with anti-windup D : Subsystem  DialogController=POWERSYS.PowerSysDialog  mask(Discrete PI Controller){Kp=Kp_Ireg, Ki=Ki_Ireg, Par_Limits=Limits_Ireg, Init=0, Ts=Ts}
      mask prompts: Kp "Proportional gain (Kp):"; Ki "Integral gain (Ki):"; Par_Limits "Output limits: [ Upper   Lower ]"; Init "Output initial value:"; Ts "Sample time:"
      mask help: This block implements a discrete PI controller.
      mask init:
      | UpperLimit=Par_Limits(1);
      | LowerLimit=Par_Limits(2);
      | power_initmask();
      mask Help: This block is part of a subset of blocks in the Extras library that does not have documentation associated with it, other than the block mask description.
      mask Display: disp('PI');
  Rtot_pu1 : Gain  Gain=Rff  SaturateOnIntegerOverflow=on  OutDataTypeStr=Inherit: Same as input  ParamDataTypeStr=Inherit: Same as input
  Rtot_pu5 : Gain  Gain=Rff  SaturateOnIntegerOverflow=on  OutDataTypeStr=Inherit: Same as input  ParamDataTypeStr=Inherit: Same as input
  Saturation : Saturate  UpperLimit=Limits_Ireg(1)  LowerLimit=Limits_Ireg(2)
  Sum : Sum  Inputs=|-+
  VdVq_conv : Outport  VectorParamsAs1DForOutWhenUnconnected=off
  PIdq : Outport  Port=2  VectorParamsAs1DForOutWhenUnconnected=off
  wires:
  Mux/1 -> Add2/2
  PI regulator with anti-windup D/1(Out) -> PIdq/1, Add2/1  "PI"
  Sum/1 -> PI regulator with anti-windup D/1(Error)
  IdIq_ref/1 -> Sum/2, Demux1/1
  IdIq_meas/1 -> Sum/1
  Add2/1 -> Saturation/1
  Saturation/1 -> VdVq_conv/1
  VdVq_meas/1 -> Demux/1
  Demux/1 -> Add1/1
  Rtot_pu1/1 -> Add1/2
  Demux1/1 -> Rtot_pu1/1, Ltot_pu2/1
  Ltot_pu1/1 -> Add1/3
  Demux1/2 -> Ltot_pu1/1, Rtot_pu5/1
  Rtot_pu5/1 -> Add3/2
  Ltot_pu2/1 -> Add3/3
  Add1/1 -> Mux/1  "Feedforward"
  Demux/2 -> Add3/1
  Add3/1 -> Mux/2

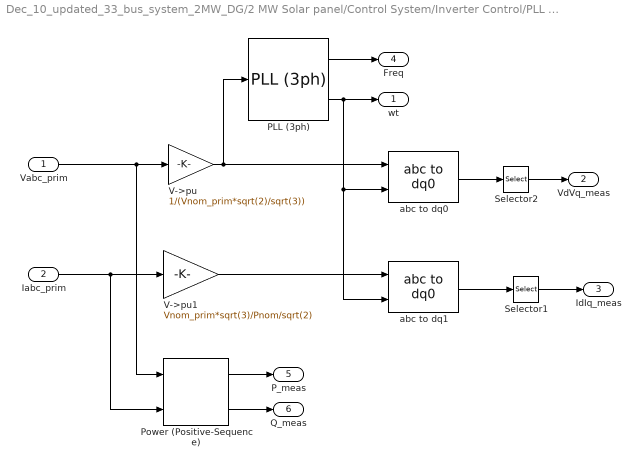
== system Dec_10_updated_33_bus_system_2MW_DG/2 MW Solar panel/Control System/Inverter Control/PLL & Measurements ==
  Vabc_prim : Inport
  Iabc_prim : Inport  Port=2
  PLL (3ph) : spsPLL3phLib/PLL (3ph)  Fmin=45  Par_Init=[-36, Fnom]  ParK=[180, 3200, 1]  TcD=1e-4  MaxRateChangeFreq=12  FilterCutOffFreq=25  Ts=Ts  AGC=off
  Power (Positive-Sequence) : spsPowerPositiveSequenceLib/Power (Positive-Sequence)  Freq=Fnom  Vinit=[20570,-37]  Iinit=[70, -63]  Ts=Ts
      settings: LibrarySourceBlock=|
      | sps_lib/Sensors and Measurements/Power
      | (Positive-Sequence)
  Selector1 : Selector  InputPortWidth=3  IndexOptions=Index vector (dialog)  Indices=[1 2]  OutputSizes=1
  Selector2 : Selector  InputPortWidth=3  IndexOptions=Index vector (dialog)  Indices=[1 2]  OutputSizes=1
  V->pu : Gain  Gain=1/(Vnom_prim*sqrt(2)/sqrt(3))  SaturateOnIntegerOverflow=on  OutDataTypeStr=Inherit: Same as input  ParamDataTypeStr=Inherit: Same as input
  V->pu1 : Gain  Gain=Vnom_prim*sqrt(3)/Pnom/sqrt(2)  SaturateOnIntegerOverflow=on  OutDataTypeStr=Inherit: Same as input  ParamDataTypeStr=Inherit: Same as input
  abc to dq0 : spsabctodq0Lib/abc to dq0  Alignment=90 degrees behind phase A axis
  abc to dq1 : spsabctodq0Lib/abc to dq0  Alignment=90 degrees behind phase A axis
  wt : Outport  VectorParamsAs1DForOutWhenUnconnected=off
  VdVq_meas : Outport  Port=2  VectorParamsAs1DForOutWhenUnconnected=off
  IdIq_meas : Outport  Port=3  VectorParamsAs1DForOutWhenUnconnected=off
  Freq : Outport  Port=4  VectorParamsAs1DForOutWhenUnconnected=off
  P_meas : Outport  Port=5  VectorParamsAs1DForOutWhenUnconnected=off
  Q_meas : Outport  Port=6  VectorParamsAs1DForOutWhenUnconnected=off
  wires:
  Power (Positive-Sequence)/2 -> Q_meas/1
  Power (Positive-Sequence)/1 -> P_meas/1
  V->pu1/1 -> abc to dq1/1
  V->pu/1 -> PLL (3ph)/1, abc to dq0/1
  abc to dq1/1 -> Selector1/1
  Vabc_prim/1 -> V->pu/1, Power (Positive-Sequence)/1
  Iabc_prim/1 -> V->pu1/1, Power (Positive-Sequence)/2
  abc to dq0/1 -> Selector2/1
  Selector2/1 -> VdVq_meas/1
  Selector1/1 -> IdIq_meas/1
  PLL (3ph)/2 -> wt/1, abc to dq1/2, abc to dq0/2
  PLL (3ph)/1 -> Freq/1

== system Dec_10_updated_33_bus_system_2MW_DG/2 MW Solar panel/Control System/Inverter Control/Reactive Power Regulator ==
  Qmeas : Inport  PortDimensions=1
  Qref : Inport  Port=2  PortDimensions=1
  On : Inport  Port=3  PortDimensions=1
  Constant1 : Constant  Value=0
  Constant2 : Constant
  PI regulator with anti-windup D : Subsystem  DialogController=POWERSYS.PowerSysDialog  mask(Discrete PI Controller){Kp=Kp_Preg, Ki=Ki_Preg, Par_Limits=Limits_Qreg, Init=0, Ts=Ts}
      mask prompts: Kp "Proportional gain (Kp):"; Ki "Integral gain (Ki):"; Par_Limits "Output limits: [ Upper   Lower ]"; Init "Output initial value:"; Ts "Sample time:"
      mask help: This block implements a discrete PI controller.
      mask init:
      | UpperLimit=Par_Limits(1);
      | LowerLimit=Par_Limits(2);
      | power_initmask();
      mask Help: This block is part of a subset of blocks in the Extras library that does not have documentation associated with it, other than the block mask description.
      mask Display: disp('PI');
  Sum : Sum  Inputs=|+-
  Switch : Switch  Criteria=u2 ~= 0  SaturateOnIntegerOverflow=off  InputSameDT=off
  W->pu1 : Gain  Gain=1/Pnom  SaturateOnIntegerOverflow=on  OutDataTypeStr=Inherit: Same as input  ParamDataTypeStr=Inherit: Same as input
  Iq_ref : Outport  InitialOutput=0  VectorParamsAs1DForOutWhenUnconnected=off
  wires:
  Qmeas/1 -> Sum/1
  Qref/1 -> Sum/2
  PI regulator with anti-windup D/1(Out) -> Iq_ref/1
  Sum/1 -> W->pu1/1
  W->pu1/1 -> PI regulator with anti-windup D/1(Error)
  Constant2/1 -> Switch/3
  Switch/1 -> PI regulator with anti-windup D/2(Reset)
  On/1 -> Switch/2
  Constant1/1 -> Switch/1

== system Dec_10_updated_33_bus_system_2MW_DG/2 MW Solar panel/Control System/Inverter Control/VDC Regulator ==
  Vdc_meas : Inport  PortDimensions=1
  Vdc_ref : Inport  Port=2  PortDimensions=1
  Kp : Inport  Port=3  PortDimensions=1
  Ki : Inport  Port=4  PortDimensions=1
  PI regulator with anti-windup D : Subsystem  DialogController=POWERSYS.PowerSysDialog  mask(Discrete PI Controller){Kp=Kp_VDCreg, Ki=Ki_VDCreg, Par_Limits=Limits_VDCreg, Init=0, Ts=Ts}
      mask prompts: Kp "Proportional gain (Kp):"; Ki "Integral gain (Ki):"; Par_Limits "Output limits: [ Upper   Lower ]"; Init "Output initial value:"; Ts "Sample time:"
      mask help: This block implements a discrete PI controller.
      mask init:
      | UpperLimit=Par_Limits(1);
      | LowerLimit=Par_Limits(2);
      | power_initmask();
      mask Help: This block is part of a subset of blocks in the Extras library that does not have documentation associated with it, other than the block mask description.
      mask Display: disp('PI');
  Rtot_pu3 : Gain  Gain=1/Vnom_dc  SaturateOnIntegerOverflow=on  OutDataTypeStr=Inherit: Same as input  ParamDataTypeStr=Inherit: Same as input
  Sum : Sum  Inputs=|+-
  Id_ref : Outport  SampleTime=Ts  InitialOutput=0  VectorParamsAs1DForOutWhenUnconnected=off
  wires:
  Ki/1 -> PI regulator with anti-windup D/3(Ki)
  Kp/1 -> PI regulator with anti-windup D/2(Kp)
  Sum/1 -> Rtot_pu3/1
  Vdc_meas/1 -> Sum/1
  Vdc_ref/1 -> Sum/2
  Rtot_pu3/1 -> PI regulator with anti-windup D/1(Error)
  PI regulator with anti-windup D/1(Out) -> Id_ref/1

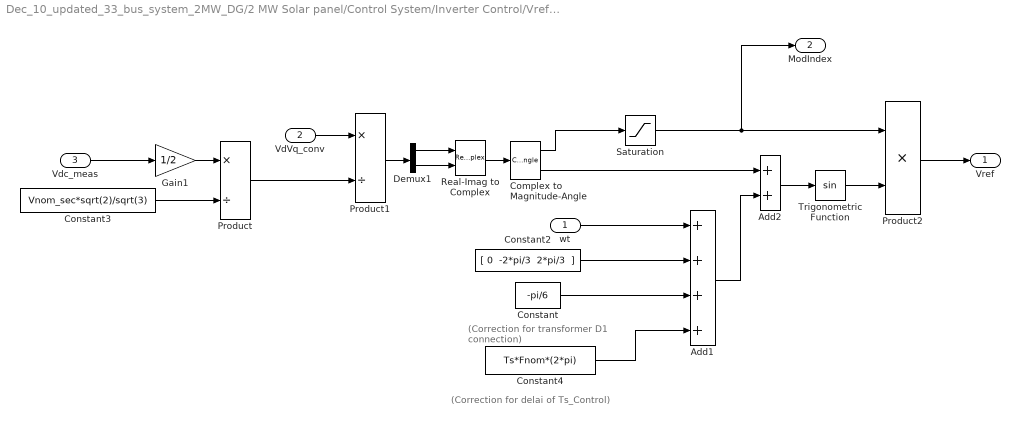
== system Dec_10_updated_33_bus_system_2MW_DG/2 MW Solar panel/Control System/Inverter Control/Vref Generation ==
  note: (Correction for transformer
      |  D1 connection)
  note: (Correction for delai of Ts_Control)
  wt : Inport
  VdVq_conv : Inport  Port=2
  Vdc_meas : Inport  Port=3
  Add1 : Sum  Inputs=++++
  Add2 : Sum
  Complex to Magnitude-Angle : ComplexToMagnitudeAngle
  Constant : Constant  Value=-pi/6
  Constant2 : Constant  Value="[ 0  -2*pi/3  2*pi/3  ]"
  Constant3 : Constant  Value=Vnom_sec*sqrt(2)/sqrt(3)
  Constant4 : Constant  Value=Ts*Fnom*(2*pi)
  Demux1 : Demux  Outputs=2
  Gain1 : Gain  Gain=1/2
  Product : Product  Inputs=*/  RndMeth=Zero
  Product1 : Product  Inputs=*/  RndMeth=Zero
  Product2 : Product  Inputs=**  RndMeth=Zero
  Real-Imag to Complex : RealImagToComplex
  Saturation : Saturate  UpperLimit=1  LowerLimit=0
  Trigonometric Function : Trigonometry
  Vref : Outport  VectorParamsAs1DForOutWhenUnconnected=off
  ModIndex : Outport  Port=2  VectorParamsAs1DForOutWhenUnconnected=off
  wires:
  Complex to Magnitude-Angle/1 -> Saturation/1
  Vdc_meas/1 -> Gain1/1
  VdVq_conv/1 -> Product1/1
  Product1/1 -> Demux1/1
  Gain1/1 -> Product/1
  Real-Imag to Complex/1 -> Complex to Magnitude-Angle/1
  Demux1/1 -> Real-Imag to Complex/1
  Demux1/2 -> Real-Imag to Complex/2
  Constant2/1 -> Add1/2
  Constant/1 -> Add1/3
  Constant3/1 -> Product/2
  Product/1 -> Product1/2
  Complex to Magnitude-Angle/2 -> Add2/1
  Add1/1 -> Add2/2
  Add2/1 -> Trigonometric Function/1
  Saturation/1 -> Product2/1, ModIndex/1
  Trigonometric Function/1 -> Product2/2
  Product2/1 -> Vref/1
  wt/1 -> Add1/1
  Constant4/1 -> Add1/4

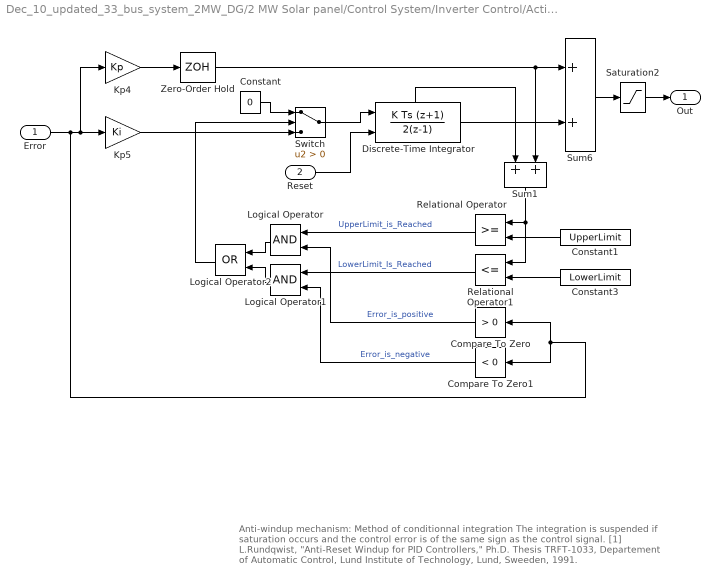
== system Dec_10_updated_33_bus_system_2MW_DG/2 MW Solar panel/Control System/Inverter Control/Active Power Regulator/PI regulator with anti-windup D ==
  note: Anti-windup mechanism: Method of conditionnal integration
      |
      | The integration is suspended if saturation occurs and the
      | control error is of the same sign as the control signal.
      |
      | [1] L.Rundqwist, "Anti-Reset Windup for PID Controllers," Ph.D. Thesis TRFT-1033,
      | Departement of Automatic Control, Lund Institute of Technology, Lund, Sweeden, 1991.
  Error : Inport  SampleTime=Ts
  Reset : Inport  Port=2  SampleTime=Ts
  Compare To Zero : simulink/Logic and Bit Operations/Compare To Zero  relop=>  OutDataTypeStr=uint8  ZeroCross=off
  Compare To Zero1 : simulink/Logic and Bit Operations/Compare To Zero  relop=<  OutDataTypeStr=uint8  ZeroCross=off
  Constant : Constant  Value=0
  Constant1 : Constant  Value=UpperLimit
  Constant3 : Constant  Value=LowerLimit
  Discrete-Time Integrator : DiscreteIntegrator  IntegratorMethod=Integration: Trapezoidal  ExternalReset=level  InitialCondition=Init  SampleTime=Ts  LimitOutput=on  UpperSaturationLimit=UpperLimit  LowerSaturationLimit=LowerLimit  ShowStatePort=on  ICPrevOutput=DiscIntNeverNeededParam  ICPrevScaledInput=DiscIntNeverNeededParam
  Kp4 : Gain  Gain=Kp  SaturateOnIntegerOverflow=on  SampleTime=Ts  OutDataTypeStr=Inherit: Same as input  ParamDataTypeStr=Inherit: Same as input
  Kp5 : Gain  Gain=Ki  SaturateOnIntegerOverflow=on  SampleTime=Ts  OutDataTypeStr=Inherit: Same as input  ParamDataTypeStr=Inherit: Same as input
  Logical Operator : Logic  AllPortsSameDT=off  OutDataTypeStr=boolean
  Logical Operator1 : Logic  AllPortsSameDT=off  OutDataTypeStr=boolean
  Logical Operator2 : Logic  Operator=OR  AllPortsSameDT=off  OutDataTypeStr=boolean
  Relational Operator : RelationalOperator  OutDataTypeStr=boolean  InputSameDT=off
  Relational Operator1 : RelationalOperator  Operator=<=  OutDataTypeStr=boolean  InputSameDT=off
  Saturation2 : Saturate  UpperLimit=UpperLimit  LowerLimit=LowerLimit  SampleTime=Ts
  Sum1 : Sum  InputSameDT=on  SaturateOnIntegerOverflow=on  SampleTime=Ts  OutDataTypeStr=Inherit: Same as first input
  Sum6 : Sum  InputSameDT=on  SaturateOnIntegerOverflow=on  SampleTime=Ts  OutDataTypeStr=Inherit: Same as first input
  Switch : Switch  Criteria=u2 > Threshold  SaturateOnIntegerOverflow=off  InputSameDT=off
  Zero-Order Hold : ZeroOrderHold  SampleTime=Ts
  Out : Outport  SampleTime=Ts  InitialOutput=0  VectorParamsAs1DForOutWhenUnconnected=off
  wires:
  Kp5/1 -> Switch/3
  Switch/1 -> Discrete-Time Integrator/1
  Saturation2/1 -> Out/1
  Discrete-Time Integrator/1 -> Sum6/2
  Kp4/1 -> Zero-Order Hold/1
  Sum6/1 -> Saturation2/1
  Error/1 -> Kp5/1, Kp4/1, Compare To Zero/1, Compare To Zero1/1
  Compare To Zero1/1 -> Logical Operator1/2  "Error_is_negative"
  Logical Operator1/1 -> Logical Operator2/2
  Logical Operator/1 -> Logical Operator2/1
  Compare To Zero/1 -> Logical Operator/2  "Error_is_positive"
  Constant3/1 -> Relational Operator1/2
  Constant1/1 -> Relational Operator/2
  Relational Operator1/1 -> Logical Operator1/1  "LowerLimit_Is_Reached"
  Relational Operator/1 -> Logical Operator/1  "UpperLimit_is_Reached"
  Logical Operator2/1 -> Switch/2
  Sum1/1 -> Relational Operator/1, Relational Operator1/1
  Discrete-Time Integrator/State -> Sum1/1
  Zero-Order Hold/1 -> Sum6/1, Sum1/2
  Constant/1 -> Switch/1
  Reset/1 -> Discrete-Time Integrator/2

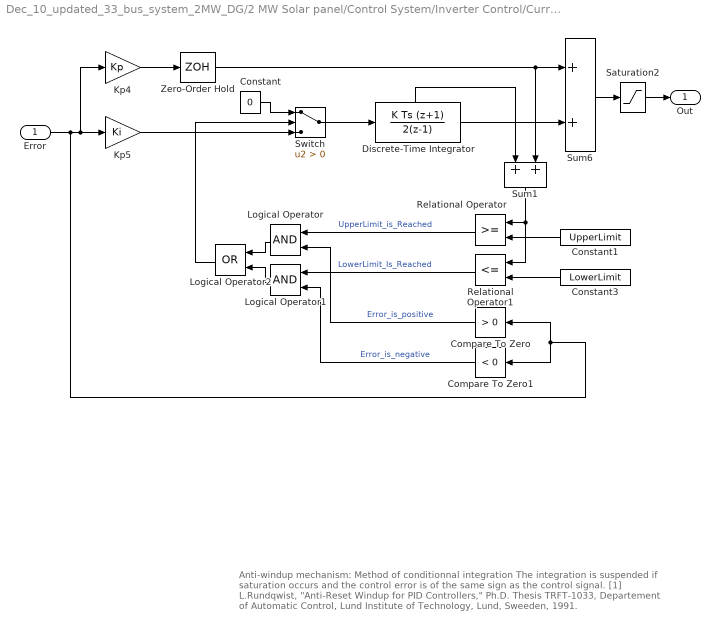
== system Dec_10_updated_33_bus_system_2MW_DG/2 MW Solar panel/Control System/Inverter Control/Current Regulator/PI regulator with anti-windup D ==
  note: Anti-windup mechanism: Method of conditionnal integration
      |
      | The integration is suspended if saturation occurs and the
      | control error is of the same sign as the control signal.
      |
      | [1] L.Rundqwist, "Anti-Reset Windup for PID Controllers," Ph.D. Thesis TRFT-1033,
      | Departement of Automatic Control, Lund Institute of Technology, Lund, Sweeden, 1991.
  Error : Inport  SampleTime=Ts
  Compare To Zero : simulink/Logic and Bit Operations/Compare To Zero  relop=>  OutDataTypeStr=uint8  ZeroCross=off
  Compare To Zero1 : simulink/Logic and Bit Operations/Compare To Zero  relop=<  OutDataTypeStr=uint8  ZeroCross=off
  Constant : Constant  Value=0
  Constant1 : Constant  Value=UpperLimit
  Constant3 : Constant  Value=LowerLimit
  Discrete-Time Integrator : DiscreteIntegrator  IntegratorMethod=Integration: Trapezoidal  InitialCondition=Init  SampleTime=Ts  LimitOutput=on  UpperSaturationLimit=UpperLimit  LowerSaturationLimit=LowerLimit  ShowStatePort=on  ICPrevOutput=DiscIntNeverNeededParam  ICPrevScaledInput=DiscIntNeverNeededParam
  Kp4 : Gain  Gain=Kp  SaturateOnIntegerOverflow=on  SampleTime=Ts  OutDataTypeStr=Inherit: Same as input  ParamDataTypeStr=Inherit: Same as input
  Kp5 : Gain  Gain=Ki  SaturateOnIntegerOverflow=on  SampleTime=Ts  OutDataTypeStr=Inherit: Same as input  ParamDataTypeStr=Inherit: Same as input
  Logical Operator : Logic  AllPortsSameDT=off  OutDataTypeStr=boolean
  Logical Operator1 : Logic  AllPortsSameDT=off  OutDataTypeStr=boolean
  Logical Operator2 : Logic  Operator=OR  AllPortsSameDT=off  OutDataTypeStr=boolean
  Relational Operator : RelationalOperator  OutDataTypeStr=boolean  InputSameDT=off
  Relational Operator1 : RelationalOperator  Operator=<=  OutDataTypeStr=boolean  InputSameDT=off
  Saturation2 : Saturate  UpperLimit=UpperLimit  LowerLimit=LowerLimit  SampleTime=Ts
  Sum1 : Sum  InputSameDT=on  SaturateOnIntegerOverflow=on  SampleTime=Ts  OutDataTypeStr=Inherit: Same as first input
  Sum6 : Sum  InputSameDT=on  SaturateOnIntegerOverflow=on  SampleTime=Ts  OutDataTypeStr=Inherit: Same as first input
  Switch : Switch  Criteria=u2 > Threshold  SaturateOnIntegerOverflow=off  InputSameDT=off
  Zero-Order Hold : ZeroOrderHold  SampleTime=Ts
  Out : Outport  SampleTime=Ts  InitialOutput=0  VectorParamsAs1DForOutWhenUnconnected=off
  wires:
  Kp5/1 -> Switch/3
  Switch/1 -> Discrete-Time Integrator/1
  Saturation2/1 -> Out/1
  Discrete-Time Integrator/1 -> Sum6/2
  Kp4/1 -> Zero-Order Hold/1
  Sum6/1 -> Saturation2/1
  Error/1 -> Kp5/1, Kp4/1, Compare To Zero/1, Compare To Zero1/1
  Compare To Zero1/1 -> Logical Operator1/2  "Error_is_negative"
  Logical Operator1/1 -> Logical Operator2/2
  Logical Operator/1 -> Logical Operator2/1
  Compare To Zero/1 -> Logical Operator/2  "Error_is_positive"
  Constant3/1 -> Relational Operator1/2
  Constant1/1 -> Relational Operator/2
  Relational Operator1/1 -> Logical Operator1/1  "LowerLimit_Is_Reached"
  Relational Operator/1 -> Logical Operator/1  "UpperLimit_is_Reached"
  Logical Operator2/1 -> Switch/2
  Sum1/1 -> Relational Operator/1, Relational Operator1/1
  Discrete-Time Integrator/State -> Sum1/1
  Zero-Order Hold/1 -> Sum6/1, Sum1/2
  Constant/1 -> Switch/1

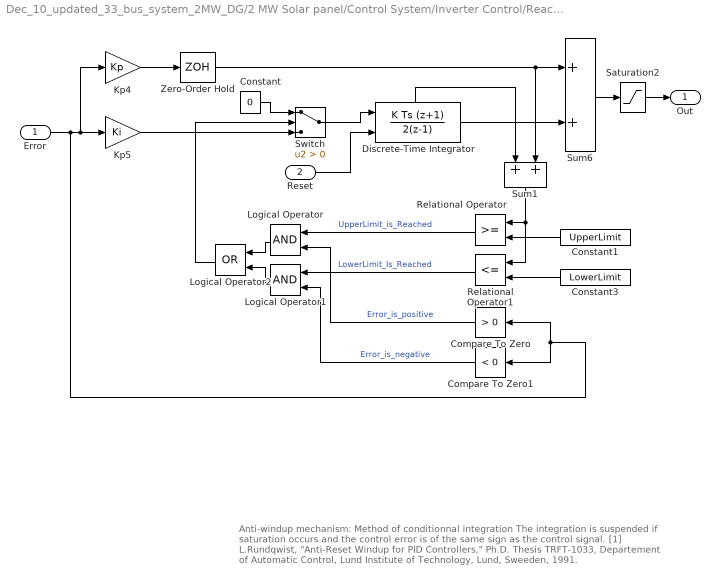
== system Dec_10_updated_33_bus_system_2MW_DG/2 MW Solar panel/Control System/Inverter Control/Reactive Power Regulator/PI regulator with anti-windup D ==
  note: Anti-windup mechanism: Method of conditionnal integration
      |
      | The integration is suspended if saturation occurs and the
      | control error is of the same sign as the control signal.
      |
      | [1] L.Rundqwist, "Anti-Reset Windup for PID Controllers," Ph.D. Thesis TRFT-1033,
      | Departement of Automatic Control, Lund Institute of Technology, Lund, Sweeden, 1991.
  Error : Inport  SampleTime=Ts
  Reset : Inport  Port=2  SampleTime=Ts
  Compare To Zero : simulink/Logic and Bit Operations/Compare To Zero  relop=>  OutDataTypeStr=uint8  ZeroCross=off
  Compare To Zero1 : simulink/Logic and Bit Operations/Compare To Zero  relop=<  OutDataTypeStr=uint8  ZeroCross=off
  Constant : Constant  Value=0
  Constant1 : Constant  Value=UpperLimit
  Constant3 : Constant  Value=LowerLimit
  Discrete-Time Integrator : DiscreteIntegrator  IntegratorMethod=Integration: Trapezoidal  ExternalReset=level  InitialCondition=Init  SampleTime=Ts  LimitOutput=on  UpperSaturationLimit=UpperLimit  LowerSaturationLimit=LowerLimit  ShowStatePort=on  ICPrevOutput=DiscIntNeverNeededParam  ICPrevScaledInput=DiscIntNeverNeededParam
  Kp4 : Gain  Gain=Kp  SaturateOnIntegerOverflow=on  SampleTime=Ts  OutDataTypeStr=Inherit: Same as input  ParamDataTypeStr=Inherit: Same as input
  Kp5 : Gain  Gain=Ki  SaturateOnIntegerOverflow=on  SampleTime=Ts  OutDataTypeStr=Inherit: Same as input  ParamDataTypeStr=Inherit: Same as input
  Logical Operator : Logic  AllPortsSameDT=off  OutDataTypeStr=boolean
  Logical Operator1 : Logic  AllPortsSameDT=off  OutDataTypeStr=boolean
  Logical Operator2 : Logic  Operator=OR  AllPortsSameDT=off  OutDataTypeStr=boolean
  Relational Operator : RelationalOperator  OutDataTypeStr=boolean  InputSameDT=off
  Relational Operator1 : RelationalOperator  Operator=<=  OutDataTypeStr=boolean  InputSameDT=off
  Saturation2 : Saturate  UpperLimit=UpperLimit  LowerLimit=LowerLimit  SampleTime=Ts
  Sum1 : Sum  InputSameDT=on  SaturateOnIntegerOverflow=on  SampleTime=Ts  OutDataTypeStr=Inherit: Same as first input
  Sum6 : Sum  InputSameDT=on  SaturateOnIntegerOverflow=on  SampleTime=Ts  OutDataTypeStr=Inherit: Same as first input
  Switch : Switch  Criteria=u2 > Threshold  SaturateOnIntegerOverflow=off  InputSameDT=off
  Zero-Order Hold : ZeroOrderHold  SampleTime=Ts
  Out : Outport  SampleTime=Ts  InitialOutput=0  VectorParamsAs1DForOutWhenUnconnected=off
  wires:
  Kp5/1 -> Switch/3
  Switch/1 -> Discrete-Time Integrator/1
  Saturation2/1 -> Out/1
  Discrete-Time Integrator/1 -> Sum6/2
  Kp4/1 -> Zero-Order Hold/1
  Sum6/1 -> Saturation2/1
  Error/1 -> Kp5/1, Kp4/1, Compare To Zero/1, Compare To Zero1/1
  Compare To Zero1/1 -> Logical Operator1/2  "Error_is_negative"
  Logical Operator1/1 -> Logical Operator2/2
  Logical Operator/1 -> Logical Operator2/1
  Compare To Zero/1 -> Logical Operator/2  "Error_is_positive"
  Constant3/1 -> Relational Operator1/2
  Constant1/1 -> Relational Operator/2
  Relational Operator1/1 -> Logical Operator1/1  "LowerLimit_Is_Reached"
  Relational Operator/1 -> Logical Operator/1  "UpperLimit_is_Reached"
  Logical Operator2/1 -> Switch/2
  Sum1/1 -> Relational Operator/1, Relational Operator1/1
  Discrete-Time Integrator/State -> Sum1/1
  Zero-Order Hold/1 -> Sum6/1, Sum1/2
  Constant/1 -> Switch/1
  Reset/1 -> Discrete-Time Integrator/2
